simulink model "ros_line_follower"  (R2021a)
settings: Solver=FixedStepDiscrete  StartTime=0.0  StopTime=inf  FixedStep=0.05  RelTol=1e-3
model workspace (MAT data in the model file):
  SL_ROS_VariableLengthArrays_MaxSizes.CommonInfo.ArrayTruncateAction = 'EmitWarning'
  SL_ROS_VariableLengthArrays_MaxSizes.MsgTypeMap = containers.Map
  SL_ROS_VariableLengthArrays_MaxSizes.MsgTypeMap.serialization.keys = {'sensor_msgs/Image'}
  SL_ROS_VariableLengthArrays_MaxSizes.MsgTypeMap.serialization.values{1}(1).PropertyName = 'Data'
  SL_ROS_VariableLengthArrays_MaxSizes.MsgTypeMap.serialization.values{1}(1).DataType = 'uint8'
  SL_ROS_VariableLengthArrays_MaxSizes.MsgTypeMap.serialization.values{1}(1).MaxLength = 2764800
  SL_ROS_VariableLengthArrays_MaxSizes.MsgTypeMap.serialization.values{1}(2).PropertyName = 'Encoding'
  SL_ROS_VariableLengthArrays_MaxSizes.MsgTypeMap.serialization.values{1}(2).DataType = 'uint8'
  SL_ROS_VariableLengthArrays_MaxSizes.MsgTypeMap.serialization.values{1}(2).MaxLength = 921600
  SL_ROS_VariableLengthArrays_MaxSizes.MsgTypeMap.serialization.uniformity = 0
  SL_ROS_VariableLengthArrays_MaxSizes.MsgTypeMap.serialization.keyType = 'char'
  SL_ROS_VariableLengthArrays_MaxSizes.MsgTypeMap.serialization.valueType = 'any'
libraries: robotlib x5, simulink x2, pid_lib x1
settings Model: EnablePacing=on  Creator=The MathWorks, Inc.  LastModifiedBy=tkikawad
settings SolverCC: AlgebraicLoopSolver=TrustRegion
settings DataIOCC: ReturnWorkspaceOutputs=off
settings OptimizationCC: LifeSpan=inf  MaxStackSize=64  EfficientTunableParamExpr=on
settings DebuggingCC: ParameterPrecisionLossMsg=none  ParameterTunabilityLossMsg=error  PregeneratedLibrarySubsystemCodeDiagnostic=none  SFExecutionAtInitializationDiag=none  SFMachineParentedDataDiag=warning  ArithmeticOperatorsInVariantConditions=warning
settings HardwareCC: ProdBitPerLong=64  ProdHWDeviceType=Intel->x86-64 (Linux 64)
settings SFSimCC: SimUseLocalCustomCode=off  MATLABDynamicMemAlloc=off  CustomCodeUndefinedFunction=UseInterfaceOnly  SimTargetLang=C++
settings RTWCC: SystemTargetFile=ert.tlc  HardwareBoard=Robot Operating System (ROS)  TLCOptions="-aInlineSetEventsForThisBaseRateFcn=TLC_FALSE -aSuppressMultiTaskScheduler=TLC_FALSE  -aRateBasedStepFcn=0"  TemplateMakefile=ert_default_tmf  GenerateReport=on  RTWUseLocalCustomCode=off  Toolchain=Catkin  IncludeHyperlinkInReport=on  LaunchReport=on  TargetLang=C++  GenerateTraceInfo=on  GenerateTraceReport=on  GenerateTraceReportSl=on  GenerateTraceReportSf=on  GenerateTraceReportEml=on  GenerateWebview=on
settings CodeAppCC: ForceParamTrailComments=on  IgnoreCustomStorageClasses=off  OperatorAnnotations=on  SimulinkDataObjDesc=on  SFDataObjDesc=on  MATLABFcnDesc=on  InsertBlockDesc=on  StateflowObjectComments=on  MATLABSourceComments=on
settings ERTTargetCC: TargetLangStandard=C99 (ISO)  MultiwordLength=2048  SupportVariableSizeSignals=on
settings ConfigComp: CovMetricSettings=dsw  CovSaveCumulativeToWorkspaceVar=on  CovSaveSingleToWorkspaceVar=on  CovExternalEMLEnable=off
settings SimscapeCC: SimscapeNormalizeSystem=off

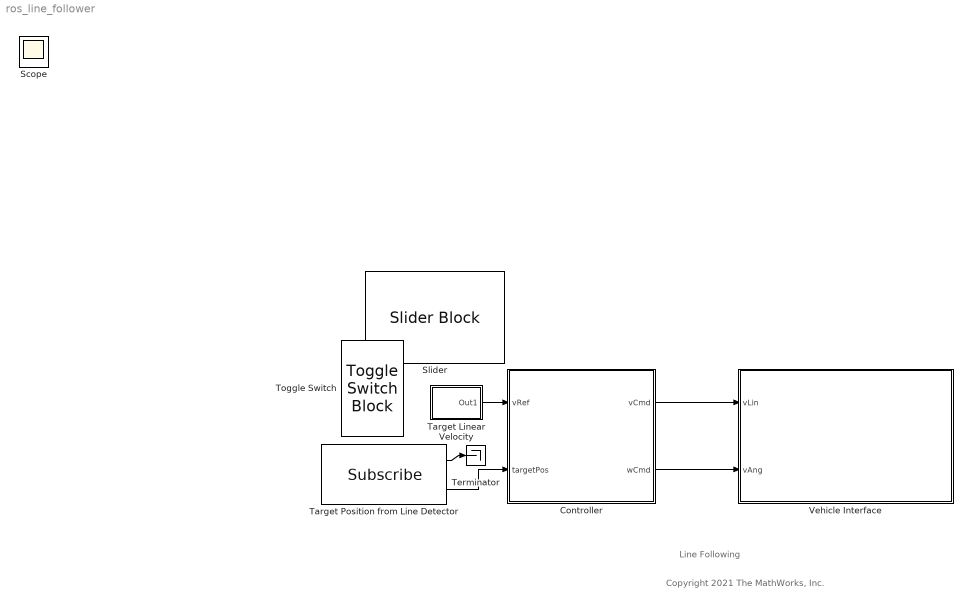
== system ros_line_follower ==
  note: Copyright 2021 The MathWorks, Inc.
  note: Line Following
  Controller : Subsystem
  Slider : SliderBlock  ScaleMax=1
  Target Linear Velocity : Subsystem
  Target Position from Line Detector : robotlib/Subscribe  topicSource=Specify your own  topic=/detection_pos  messageType=std_msgs/Float32MultiArray  SampleTime=0.1  legacyBusStruct=off  messageQueueLength=1
  Terminator : Terminator
  Toggle Switch : ToggleSwitchBlock
      settings: Values={{'Off', 'On'}, [0 1]}
  Vehicle Interface : Subsystem
  Scope : Scope
  wires:
  Controller/1(vCmd) -> Vehicle Interface/1(vLin)
  Controller/2(wCmd) -> Vehicle Interface/2(vAng)
  Target Position from Line Detector/2 -> Controller/2(targetPos)
  Target Position from Line Detector/1 -> Terminator/1
  Target Linear Velocity/1(Out1) -> Controller/1(vRef)

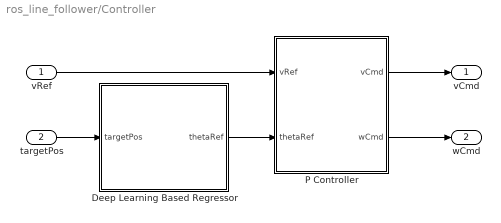
== system ros_line_follower/Controller ==
  vRef : Inport
  targetPos : Inport  Port=2
  Deep Learning Based Regressor : Subsystem
  P Controller : Subsystem
  vCmd : Outport
  wCmd : Outport  Port=2
  wires:
  P Controller/1(vCmd) -> vCmd/1
  P Controller/2(wCmd) -> wCmd/1
  targetPos/1 -> Deep Learning Based Regressor/1(targetPos)
  vRef/1 -> P Controller/1(vRef)
  Deep Learning Based Regressor/1(thetaRef) -> P Controller/2(thetaRef)

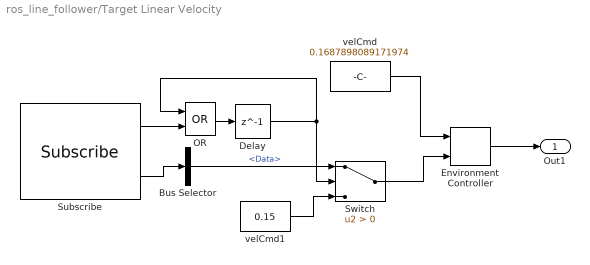
== system ros_line_follower/Target Linear Velocity ==
  Bus Selector : BusSelector  OutputSignals=Data
  Delay : Delay  DelayLength=1
  Environment Controller : simulink/Signal Routing/Environment Controller
      settings: SourceProductBaseCode=SL
  OR : Logic  Operator=OR  AllPortsSameDT=off  OutDataTypeStr=boolean
  Subscribe : robotlib/Subscribe  topicSource=Specify your own  topic=/line_follower/linear_velocity  messageType=std_msgs/Float32  SampleTime=-1  legacyBusStruct=off  messageQueueLength=1
  Switch : Switch  Criteria=u2 > Threshold
  velCmd : Constant  Value=0.1687898089171974  SampleTime=-1
  velCmd1 : Constant  Value=0.15  SampleTime=-1
  Out1 : Outport
  wires:
  Bus Selector/1 -> Switch/1  "<Data>"
  OR/1 -> Delay/1
  Delay/1 -> Switch/2, OR/1
  Subscribe/2 -> Bus Selector/1
  velCmd/1 -> Environment Controller/1
  Subscribe/1 -> OR/2
  Environment Controller/1 -> Out1/1
  Switch/1 -> Environment Controller/2
  velCmd1/1 -> Switch/3

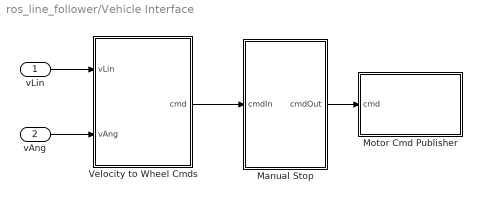
== system ros_line_follower/Vehicle Interface ==
  vLin : Inport
  vAng : Inport  Port=2
  Manual Stop : Subsystem
  Motor Cmd Publisher : Subsystem
  Velocity to Wheel Cmds : MATLAB Function  TreatAsAtomicUnit=on
  wires:
  vLin/1 -> Velocity to Wheel Cmds/1(vLin)
  Manual Stop/1(cmdOut) -> Motor Cmd Publisher/1(cmd)
  Velocity to Wheel Cmds/1(cmd) -> Manual Stop/1(cmdIn)
  vAng/1 -> Velocity to Wheel Cmds/2(vAng)

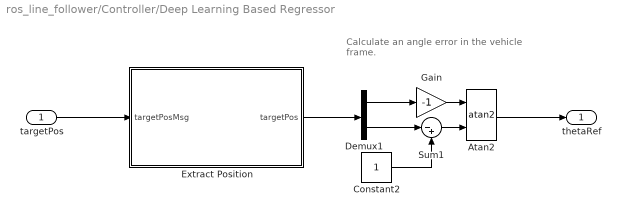
== system ros_line_follower/Controller/Deep Learning Based Regressor ==
  note: Calculate an angle error
      | in the vehicle frame.
  targetPos : Inport
  Atan2 : Trigonometry  Operator=atan2
  Constant2 : Constant  OutDataTypeStr=single
  Demux1 : Demux  Outputs=2
  Extract Position : Subsystem
  Gain : Gain  Gain=-1
  Sum1 : Sum  Inputs=|-+
  thetaRef : Outport
  wires:
  Demux1/1 -> Gain/1
  Atan2/1 -> thetaRef/1
  Demux1/2 -> Sum1/1
  Sum1/1 -> Atan2/2
  Constant2/1 -> Sum1/2
  Extract Position/1(targetPos) -> Demux1/1
  targetPos/1 -> Extract Position/1(targetPosMsg)
  Gain/1 -> Atan2/1

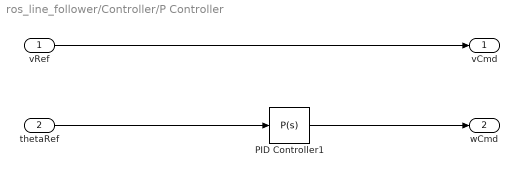
== system ros_line_follower/Controller/P Controller ==
  vRef : Inport
  thetaRef : Inport  Port=2
  PID Controller1 : pid_lib/PID Controller  Controller=P  Form=Parallel  TimeDomain=Continuous-time  UseExternalTs=off  SampleTime=0.01  IntegratorMethod=Forward Euler  FilterMethod=Forward Euler  ControllerParametersSource=internal  P=2.5  I=0.01  D=0.5  UseFilter=on  N=100  TunerSelectOption=Transfer Function Based (PID Tuner App)  InitialConditionSource=internal  InitialConditionForIntegrator=0  InitialConditionForFilter=0  DifferentiatorICPrevScaledInput=0  ExternalReset=none  TrackingMode=off  Kt=1  LimitOutput=off  SatLimitsSource=internal  UpperSaturationLimit=inf  LowerSaturationLimit=-inf  LinearizeAsGain=on  AntiWindupMode=none  Kb=1  POutMin=[]  POutMax=[]  IOutMin=[]  IOutMax=[]  DOutMin=[]  DOutMax=[]  NOutMin=[]  NOutMax=[]  SumOutMin=[]  SumOutMax=[]  SaturationOutMin=[]  SaturationOutMax=[]  PParamMin=[]  PParamMax=[]  IParamMin=[]  IParamMax=[]  DParamMin=[]  DParamMax=[]  NParamMin=[]  NParamMax=[]  KbParamMin=[]  KbParamMax=[]  KtParamMin=[]  KtParamMax=[]  KbOutMin=[]  KbOutMax=[]  KtOutMin=[]  KtOutMax=[]  IntegratorOutMin=[]  IntegratorOutMax=[]  FilterOutMin=[]  FilterOutMax=[]  SumI1OutMin=[]  SumI1OutMax=[]  SumI2OutMin=[]  SumI2OutMax=[]  SumI3OutMin=[]  SumI3OutMax=[]  SumI4OutMin=[]  SumI4OutMax=[]  SumDOutMin=[]  SumDOutMax=[]  DifferentiatorOutMin=[]  DifferentiatorOutMax=[]  FilterDiffOutCoefMin=[]  FilterDiffOutCoefMax=[]  ReciprocalOutMin=[]  ReciprocalOutMax=[]  SumDenOutMin=[]  SumDenOutMax=[]  SumNumOutMin=[]  SumNumOutMax=[]  DivideOutMin=[]  DivideOutMax=[]  UdiffTsProdOutMin=[]  UdiffTsProdOutMax=[]  NTsProdOutMin=[]  NTsProdOutMax=[]  UintegralTsProdOutMin=[]  UintegralTsProdOutMax=[]  UngainTsProdOutMin=[]  UngainTsProdOutMax=[]  IntegratorContinuousStateAttributes=''  IntegratorStateMustResolveToSignalObject=off  IntegratorRTWStateStorageClass=Auto  FilterContinuousStateAttributes=''  FilterStateMustResolveToSignalObject=off  FilterRTWStateStorageClass=Auto  ParallelPVariant=InternalParameters  IdealPVariant=Disabled  IVariant=Disabled  DVariant=Disabled  IntegratorVariant=Disabled  SatVariant=Disabled  AWVariant=Disabled  PCopyVariant=Disabled  TRVariant=Disabled  FdbkBlocksVariant=Forward  IdealPFdbkVariant=Disabled  SatFdbkVariant=Disabled  DerivativeFilterVariant=Disabled  NVariant=Disabled  NCopyVariant=Disabled_SignalSpec  FilterICVariant=Disabled  IntegratorICVariant=Disabled  ExternalResetVariant=Disabled  TRSumVariant=Passthrough  SumFdbkVariant=Disabled  SumVariant=Passthrough_P  TsampFilterVariant=InternalTs  TsampNgainVariant=Passthrough  TsampIntegralVariant=Disabled_SignalSpec  ExternalSaturationOutDataTypeStr=Inherit: Same as second input
  vCmd : Outport
  wCmd : Outport  Port=2
  wires:
  vRef/1 -> vCmd/1
  PID Controller1/1 -> wCmd/1
  thetaRef/1 -> PID Controller1/1

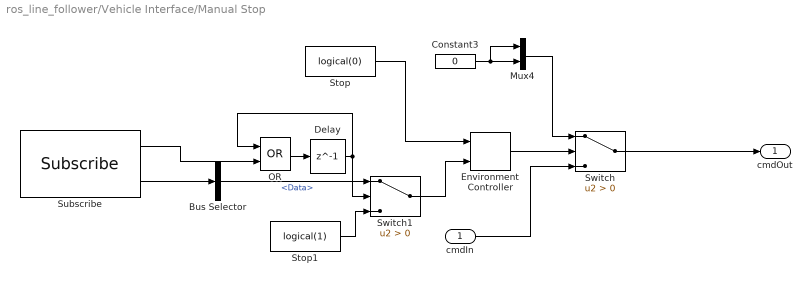
== system ros_line_follower/Vehicle Interface/Manual Stop ==
  cmdIn : Inport
  Bus Selector : BusSelector  OutputSignals=Data
  Constant3 : Constant  Value=0  OutDataTypeStr=single  SampleTime=-1
  Delay : Delay  DelayLength=1
  Environment Controller : simulink/Signal Routing/Environment Controller
      settings: SourceProductBaseCode=SL
  Mux4 : Mux  Inputs=2
  OR : Logic  Operator=OR  AllPortsSameDT=off  OutDataTypeStr=boolean
  Stop : Constant  Value=logical(0)  SampleTime=-1
  Stop1 : Constant  Value=logical(1)  SampleTime=-1
  Subscribe : robotlib/Subscribe  topicSource=Specify your own  topic=/line_follower/stop  messageType=std_msgs/Bool  SampleTime=-1  legacyBusStruct=off  messageQueueLength=1
  Switch : Switch  Criteria=u2 > Threshold
  Switch1 : Switch  Criteria=u2 > Threshold
  cmdOut : Outport
  wires:
  Mux4/1 -> Switch/1
  Constant3/1 -> Mux4/1, Mux4/2
  cmdIn/1 -> Switch/3
  Stop/1 -> Environment Controller/1
  Switch/1 -> cmdOut/1
  Subscribe/2 -> Bus Selector/1
  Delay/1 -> Switch1/2, OR/1
  Subscribe/1 -> OR/2
  OR/1 -> Delay/1
  Bus Selector/1 -> Switch1/1  "<Data>"
  Environment Controller/1 -> Switch/2
  Stop1/1 -> Switch1/3
  Switch1/1 -> Environment Controller/2

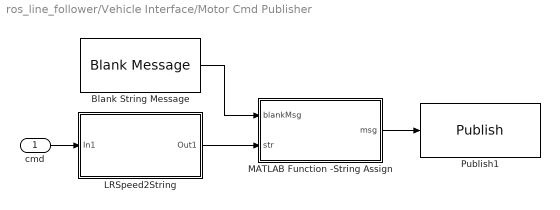
== system ros_line_follower/Vehicle Interface/Motor Cmd Publisher ==
  cmd : Inport
  Blank String Message : robotlib/Blank Message  messageClass=Message  entityType=std_msgs/String  messageType=std_msgs/String  SampleTime=inf  legacyBusStruct=off
  LRSpeed2String : Subsystem
  MATLAB Function -String Assign : MATLAB Function  TreatAsAtomicUnit=on
  Publish1 : robotlib/Publish  topicSource=Specify your own  topic=/jetbot_motors/cmd_raw  messageType=std_msgs/String  legacyBusStruct=off  messageQueueLength=1
  wires:
  MATLAB Function -String Assign/1(msg) -> Publish1/1
  Blank String Message/1 -> MATLAB Function -String Assign/1(blankMsg)
  LRSpeed2String/1(Out1) -> MATLAB Function -String Assign/2(str)
  cmd/1 -> LRSpeed2String/1(In1)

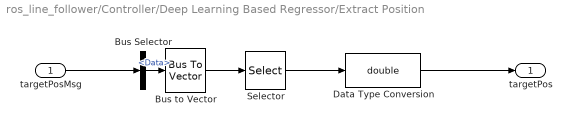
== system ros_line_follower/Controller/Deep Learning Based Regressor/Extract Position ==
  targetPosMsg : Inport
  Bus Selector : BusSelector  OutputSignals=Data
  Bus to Vector : BusToVector
  Data Type Conversion : DataTypeConversion  OutDataTypeStr=double
  Selector : Selector  InputPortWidth=128  IndexOptions=Index vector (dialog)  Indices=1:2  OutputSizes=1
  targetPos : Outport
  wires:
  targetPosMsg/1 -> Bus Selector/1
  Bus Selector/1 -> Bus to Vector/1  "<Data>"
  Bus to Vector/1 -> Selector/1
  Selector/1 -> Data Type Conversion/1
  Data Type Conversion/1 -> targetPos/1

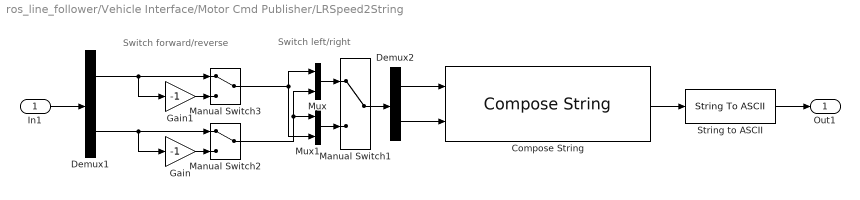
== system ros_line_follower/Vehicle Interface/Motor Cmd Publisher/LRSpeed2String ==
  note: Switch forward/reverse
  note: Switch left/right
  In1 : Inport
  Compose String : ComposeString  Format="\"speed[ %+1.4f,%+1.4f ]\""
  Demux1 : Demux  Outputs=2
  Demux2 : Demux  Outputs=2
  Gain : Gain  Gain=-1
  Gain1 : Gain  Gain=-1
  Manual Switch1 : ManualSwitch
  Manual Switch2 : ManualSwitch
  Manual Switch3 : ManualSwitch
  Mux : Mux  Inputs=2
  Mux1 : Mux  Inputs=2
  String to ASCII : StringToASCII
  Out1 : Outport  VectorParamsAs1DForOutWhenUnconnected=off
  wires:
  Manual Switch2/1 -> Mux1/1, Mux/2
  Manual Switch3/1 -> Mux1/2, Mux/1
  Mux1/1 -> Manual Switch1/2
  Mux/1 -> Manual Switch1/1
  Manual Switch1/1 -> Demux2/1
  Demux1/1 -> Manual Switch3/1, Gain1/1
  Gain1/1 -> Manual Switch3/2
  Gain/1 -> Manual Switch2/2
  Demux1/2 -> Manual Switch2/1, Gain/1
  String to ASCII/1 -> Out1/1
  Compose String/1 -> String to ASCII/1
  In1/1 -> Demux1/1
  Demux2/2 -> Compose String/2
  Demux2/1 -> Compose String/1

== matlab function ros_line_follower/Vehicle Interface/Velocity to Wheel Cmds ==
  data: vLin input; cmd output; vAng input
function cmd = vel2wheel(vLin,vAng)
%#codegen
d = 0.05125*2;
r = 0.03;

if abs(vAng) > 2
    vl = -d*vAng/2;
    vr =  d*vAng/2;
else
    vl = vLin - d*vAng/2;
    vr = vLin + d*vAng/2;
end
wl = vl / r;
wr = vr / r;
wlCmd = funcl(wl);
wrCmd = funcr(wr);
cmd = [wlCmd,wrCmd];

    function wCmd = funcl(w)
        wCmd = min(max(w*0.1,-1),1);
    end
    function wCmd = funcr(w)
        wCmd = min(max(w*0.096,-1),1);
    end
end

== matlab function ros_line_follower/Vehicle Interface/Motor Cmd Publisher/MATLAB Function -String Assign ==
  data: blankMsg input; msg output Bus: SL_Bus_ros_line_follower_std_msgs_String; str input
function msg = assignStringInput(blankMsg, str)
% assignStringInput - Assign a string in a ROS message to specified input string
%
% MSG = assignStringInput(blankMsg, STR) assigns the input string, STR, to
%  a string field in the ROS message, blankMsg, and outputs the updated
%  ROS message.
%
%  Inputs
%    blankMsg: A bus for a 'std_msgs/String' message. This is 
%        used to initialize the output.
%    str: An array of uint8 that will be assigned to the 'Data' field
%        in blankMsg. The entire array is assumed to be a valid sequence of
%        character ASCII values.
% 
%  Outputs:
%    msg: A bus for a 'std_msgs/String' message, with the 'Data'
%        field set to a string.

%   Copyright 2015 The MathWorks, Inc.
%#codegen

% Note: The datatype of 'msg' has been explicitly set to the appropriate 
% Simulink bus type ("Bus: SL_Bus_robotROSMessageUsageExample_std_msgs_String"). 
%
% If the model name is changed, the datatype needs to be changed as well:
%   1) Click "Edit Data" in the Editor toolstrip to open "Ports and Data Manager"
%   2) Select "msg". From the "Type" dropdown, select "--- Refresh data types ---"
%   3) Set datatype to "Bus: SL_Bus_<modelname>_std_msgs_String"
    
msg = blankMsg;

% msg (std_msgs/String) consists of
%           Data : array of type uint8
%   Data_SL_Info : struct with fields CurrentLength, ReceivedLength
strLength = length(str);
msg.Data(1:strLength) = uint8(str);
msg.Data_SL_Info.CurrentLength = uint32(strLength);
